simulink model "Test_CommSM"  (R2017b)
settings: Solver=VariableStepAuto  StartTime=0.0  StopTime=inf  RelTol=1e-3
model workspace (MAT data in the model file):
  AP = Simulink.Signal
  AP.DataType = 'double'
  AP.Dimensions = 1
  AP.DimensionsMode = 'auto'
  AP.Complexity = 'real'
  AP.SampleTime = -1
  AP.SamplingMode = 'auto'
  AP.InitialValue = '0'
  ZPT_1 = Simulink.Signal
  ZPT_1.DataType = 'double'
  ZPT_1.Dimensions = [1 3]
  ZPT_1.DimensionsMode = 'Fixed'
  ZPT_1.Complexity = 'real'
  ZPT_1.SampleTime = -1
  ZPT_1.SamplingMode = 'auto'
  ZPT_1.InitialValue = 'zeros(1,3)'
  ZZPT_1 = Simulink.Signal
  ZZPT_1.DataType = 'double'
  ZZPT_1.Dimensions = [3 4]
  ZZPT_1.DimensionsMode = 'Fixed'
  ZZPT_1.Complexity = 'real'
  ZZPT_1.SampleTime = -1
  ZZPT_1.SamplingMode = 'auto'
  ZZPT_1.InitialValue = 'zeros(3,4)'
settings Model: Creator=张紫薇  LastModifiedBy=张紫薇

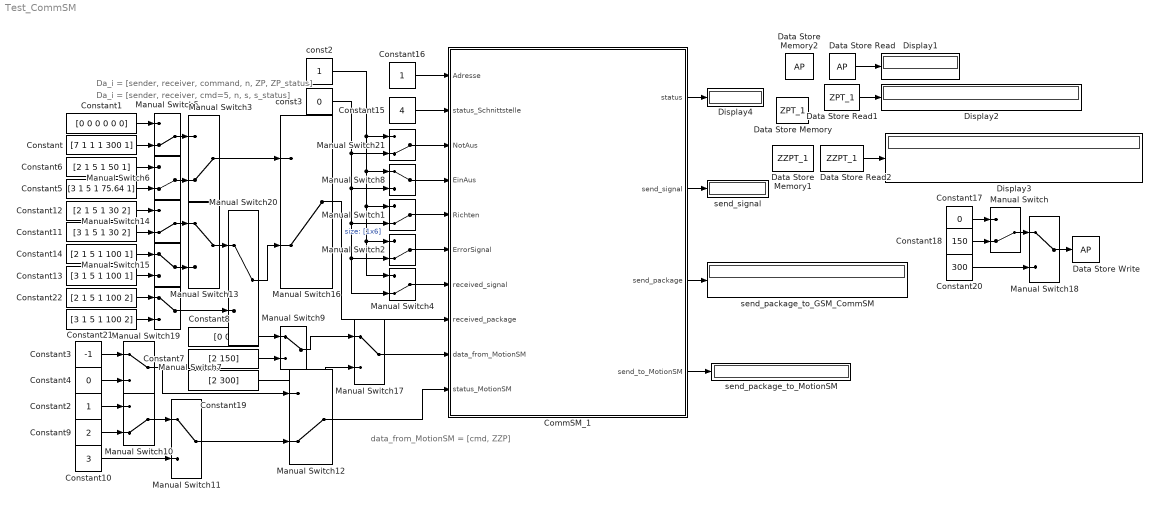
== system Test_CommSM ==
  note: data_from_MotionSM = [cmd, ZZP]
  note: Da_i = [sender, receiver, command, n, ZP, ZP_status]
  note: Da_i = [sender, receiver, cmd=5, n, s, s_status]
  CommSM_1 : Subsystem
  Constant : Constant  Value=[7 1 1 1 300 1]  OutDataTypeStr=double
  Constant1 : Constant  Value=[0 0 0 0 0 0]  OutDataTypeStr=double
  Constant10 : Constant  Value=3  OutDataTypeStr=double
  Constant11 : Constant  Value=[3 1 5 1 30 2]  OutDataTypeStr=double
  Constant12 : Constant  Value=[2 1 5 1 30 2]  OutDataTypeStr=double
  Constant13 : Constant  Value=[3 1 5 1 100 1]  OutDataTypeStr=double
  Constant14 : Constant  Value=[2 1 5 1 100 1]  OutDataTypeStr=double
  Constant15 : Constant  Value=4  OutDataTypeStr=double
  Constant16 : Constant
  Constant17 : Constant  Value=0  OutDataTypeStr=double
  Constant18 : Constant  Value=150  OutDataTypeStr=double
  Constant19 : Constant  Value=[2 300]  OutDataTypeStr=double
  Constant2 : Constant  OutDataTypeStr=double
  Constant20 : Constant  Value=300  OutDataTypeStr=double
  Constant21 : Constant  Value=[3 1 5 1 100 2]  OutDataTypeStr=double
  Constant22 : Constant  Value=[2 1 5 1 100 2]  OutDataTypeStr=double
  Constant3 : Constant  Value=-1  OutDataTypeStr=double
  Constant4 : Constant  Value=0  OutDataTypeStr=double
  Constant5 : Constant  Value=[3 1 5 1 75.64 1]  OutDataTypeStr=double
  Constant6 : Constant  Value=[2 1 5 1 50 1]  OutDataTypeStr=double
  Constant7 : Constant  Value=[2 150]  OutDataTypeStr=double
  Constant8 : Constant  Value=[0 0]  OutDataTypeStr=double
  Constant9 : Constant  Value=2  OutDataTypeStr=double
  Data Store Memory : DataStoreMemory  DataStoreName=ZPT_1  ReadBeforeWriteMsg=warning  WriteAfterWriteMsg=warning  WriteAfterReadMsg=warning  InitialValue=zeros(1,3)  ShowAdditionalParam=off  OutDataTypeStr=double  Dimensions=[1,3]
  Data Store Memory1 : DataStoreMemory  DataStoreName=ZZPT_1  ReadBeforeWriteMsg=warning  WriteAfterWriteMsg=warning  WriteAfterReadMsg=warning  InitialValue=zeros(3,4)  ShowAdditionalParam=off  OutDataTypeStr=double  Dimensions=[3,4]
  Data Store Memory2 : DataStoreMemory  DataStoreName=AP  ReadBeforeWriteMsg=warning  WriteAfterWriteMsg=warning  WriteAfterReadMsg=warning  ShowAdditionalParam=off  OutDataTypeStr=double  Dimensions=1
  Data Store Read : DataStoreRead  DataStoreName=AP
  Data Store Read1 : DataStoreRead  DataStoreName=ZPT_1
  Data Store Read2 : DataStoreRead  DataStoreName=ZZPT_1
  Data Store Write : DataStoreWrite  DataStoreName=AP
  Display{1..4} (4 alike) : Display
  Manual Switch{,1..6,10,12,14,16,21} (12 alike) : ManualSwitch  CurrentSetting=0
  Manual Switch{7..9,11,13,15,17..20} (10 alike) : ManualSwitch
  const2 : Constant  OutDataTypeStr=boolean
  const3 : Constant  Value=0  OutDataTypeStr=boolean
  send_package_to_GSM_CommSM : Display
  send_package_to_MotionSM : Display
  send_signal : Display
  wires:
  const2/1 -> Manual Switch4/1, Manual Switch2/1, Manual Switch1/1, Manual Switch8/1, Manual Switch21/1
  const3/1 -> Manual Switch21/2, Manual Switch4/2, Manual Switch2/2, Manual Switch1/2, Manual Switch8/2
  Manual Switch21/1 -> CommSM_1/3(NotAus)
  Manual Switch8/1 -> CommSM_1/4(EinAus)
  Manual Switch1/1 -> CommSM_1/5(Richten)
  Manual Switch2/1 -> CommSM_1/6(ErrorSignal)
  Manual Switch4/1 -> CommSM_1/7(received_signal)
  Manual Switch5/1 -> Manual Switch3/1
  Constant1/1 -> Manual Switch5/1
  Constant/1 -> Manual Switch5/2
  Constant6/1 -> Manual Switch6/1
  Constant5/1 -> Manual Switch6/2
  Manual Switch6/1 -> Manual Switch3/2
  Constant8/1 -> Manual Switch9/1
  Constant7/1 -> Manual Switch9/2
  Constant3/1 -> Manual Switch7/1
  Constant4/1 -> Manual Switch7/2
  Constant2/1 -> Manual Switch10/1
  Constant9/1 -> Manual Switch10/2
  Manual Switch10/1 -> Manual Switch11/1
  Constant10/1 -> Manual Switch11/2
  Manual Switch7/1 -> Manual Switch12/1
  Manual Switch11/1 -> Manual Switch12/2
  Manual Switch12/1 -> CommSM_1/10(status_MotionSM)
  Constant13/1 -> Manual Switch15/2
  Constant14/1 -> Manual Switch15/1
  Constant12/1 -> Manual Switch14/1
  Constant11/1 -> Manual Switch14/2
  Manual Switch14/1 -> Manual Switch13/1
  Manual Switch15/1 -> Manual Switch13/2
  Manual Switch3/1 -> Manual Switch16/1
  Manual Switch16/1 -> CommSM_1/8(received_package)  "size: [1x6]"
  CommSM_1/2(send_signal) -> send_signal/1
  CommSM_1/3(send_package) -> send_package_to_GSM_CommSM/1
  CommSM_1/4(send_to_MotionSM) -> send_package_to_MotionSM/1
  Constant15/1 -> CommSM_1/2(status_Schnittstelle)
  Constant16/1 -> CommSM_1/1(Adresse)
  CommSM_1/1(status) -> Display4/1
  Data Store Read2/1 -> Display3/1
  Data Store Read/1 -> Display1/1
  Data Store Read1/1 -> Display2/1
  Constant17/1 -> Manual Switch/1
  Constant18/1 -> Manual Switch/2
  Constant19/1 -> Manual Switch17/2
  Manual Switch9/1 -> Manual Switch17/1
  Manual Switch17/1 -> CommSM_1/9(data_from_MotionSM)
  Constant20/1 -> Manual Switch18/2
  Manual Switch/1 -> Manual Switch18/1
  Manual Switch18/1 -> Data Store Write/1
  Constant22/1 -> Manual Switch19/1
  Constant21/1 -> Manual Switch19/2
  Manual Switch19/1 -> Manual Switch20/2
  Manual Switch13/1 -> Manual Switch20/1
  Manual Switch20/1 -> Manual Switch16/2

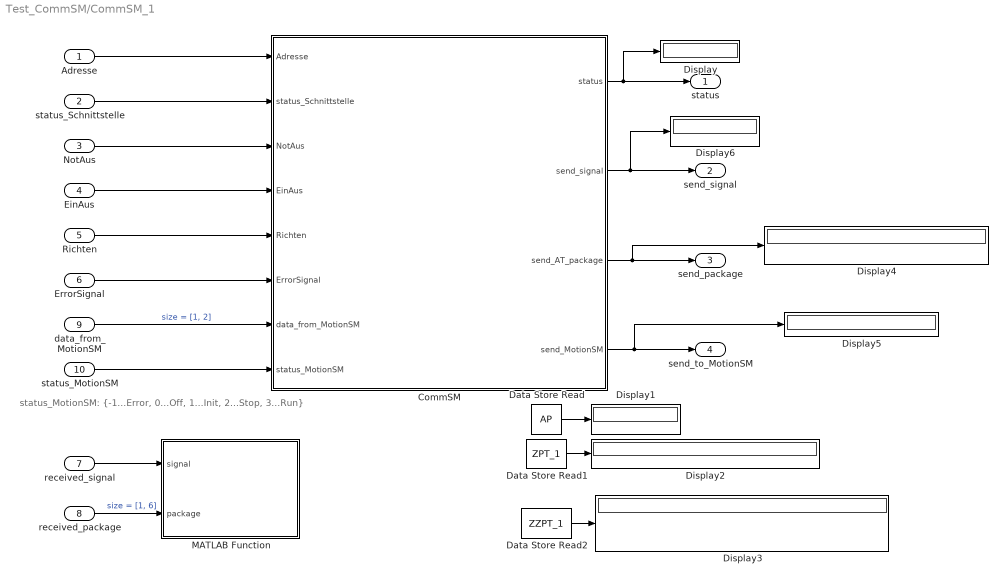
== system Test_CommSM/CommSM_1 ==
  note: status_MotionSM: {-1...Error, 0...Off, 1...Init, 2...Stop, 3...Run}
  Adresse : Inport  OutDataTypeStr=double  PortDimensions=1
  status_Schnittstelle : Inport  Port=2  OutDataTypeStr=double  PortDimensions=1
  NotAus : Inport  Port=3  OutDataTypeStr=boolean  PortDimensions=1
  EinAus : Inport  Port=4  OutDataTypeStr=boolean  PortDimensions=1
  Richten : Inport  Port=5  OutDataTypeStr=boolean  PortDimensions=1
  ErrorSignal : Inport  Port=6  OutDataTypeStr=boolean  PortDimensions=1
  received_signal : Inport  Port=7  OutDataTypeStr=boolean  PortDimensions=1
  received_package : Inport  Port=8  OutDataTypeStr=double  PortDimensions=6
  data_from_MotionSM : Inport  Port=9  OutDataTypeStr=double  PortDimensions=2
  status_MotionSM : Inport  Port=10  OutDataTypeStr=double  PortDimensions=1
  CommSM : Stateflow chart  TreatAsAtomicUnit=on
  Data Store Read : DataStoreRead  DataStoreName=AP
  Data Store Read1 : DataStoreRead  DataStoreName=ZPT_1
  Data Store Read2 : DataStoreRead  DataStoreName=ZZPT_1
  Display{,1..6} (7 alike) : Display
  MATLAB Function : MATLAB Function  TreatAsAtomicUnit=on
  status : Outport  OutDataTypeStr=double  PortDimensions=1
  send_signal : Outport  Port=2  OutDataTypeStr=boolean  PortDimensions=1
  send_package : Outport  Port=3  OutDataTypeStr=double  PortDimensions=6
  send_to_MotionSM : Outport  Port=4  OutDataTypeStr=double  PortDimensions=2
  wires:
  NotAus/1 -> CommSM/3(NotAus)
  EinAus/1 -> CommSM/4(EinAus)
  Richten/1 -> CommSM/5(Richten)
  ErrorSignal/1 -> CommSM/6(ErrorSignal)
  status_Schnittstelle/1 -> CommSM/2(status_Schnittstelle)
  received_signal/1 -> MATLAB Function/1(signal)
  received_package/1 -> MATLAB Function/2(package)  "size = [1, 6]"
  data_from_MotionSM/1 -> CommSM/7(data_from_MotionSM)  "size = [1, 2]"
  status_MotionSM/1 -> CommSM/8(status_MotionSM)
  Adresse/1 -> CommSM/1(Adresse)
  CommSM/1(status) -> Display/1, status/1
  CommSM/3(send_AT_package) -> Display4/1, send_package/1
  CommSM/4(send_MotionSM) -> Display5/1, send_to_MotionSM/1
  CommSM/2(send_signal) -> Display6/1, send_signal/1
  Data Store Read/1 -> Display1/1
  Data Store Read1/1 -> Display2/1
  Data Store Read2/1 -> Display3/1

== matlab function Test_CommSM/CommSM_1/MATLAB Function ==
  data: signal input boolean size=1; package input double size=[1,6]; ZPT_1 data_store_memory; ZZPT_1 data_store_memory
%Protokoll
%SummenTelegramm = [HDR, SDT, END]
	%HDR: header,	SDT: Summen-Daten-Telegramm,    END: Ender

%SDT = [SDT_7, SDT_1, SDT_2, SDT_3]
%SDT_i = [Da_i, De_i]
	%Da: Data, De: Delay
	%i...{1,2,3,7}	%7...GSM, 1-3...CommSM1-3

%Da_i = [sender, receiver, cmd, N, ZP, ZP_status]
	%sender,receiver...{1,2,3,7,255}	%255...Broadcast
	%cmd: 1...addP, 2...getP, 3...setS, 4...getS
	%ZP_status: 0...none, 1...wait, 2...active, 3...done, 4...error

%Da_i = [sender, receiver, cmd, N, s, s_status]
	%cmd: 5...negO
	%s_status: 0...none, 1...negotiation, 2...excute, 3...done

function receive_AT(signal, package)

global ZPT_1
global ZZPT_1

if signal
    switch package(1)  % from GSM
        case 7
            if (package(3) == 1)   % add Position
                if ZPT_1(1) == 0
                    ZPT_1 = package(4:6)';    %[n, ZP, status='wait']
                end
            end
            
        case {2,3}      % from CommSM_2 or CommSM_3
            if package(3) == 5      % negotiation
                switch package(6)
                    case 1      % nego
                        ZZPT_1(package(1),:) = [package(4), 0, package(5:6)];     % [n, ZP, s%, status='nego']
                    case 2      % excu
                        if ZZPT_1(package(1),4) == 1
                            ZZPT_1(package(1),4) = package(6);
                        end
                end
            end
    end
end

end

== stateflow chart Test_CommSM/CommSM_1/CommSM ==
  state Init
    entry: 	status=1;
    send_AT_package=[Adresse, zeros(1,5)];
    send_signal=false;
    send_MotionSM=[0,0];
  state Aus
    entry: status=0;
  state Ein
    note: % Protokoll
        | % SummenTelegramm = [HDR, SDT, END]
        | %HDR: header, SDT: Summen-Daten-Telegramm, END: Ender
        |
        | % SDT = [SDT_7, SDT_1, SDT_2, SDT_3]
        | % SDT_i = [Da_i, De_i]
        | %Da: Data, De: Delay
        | %i...{1,2,3,7} %7...GSM, 1-3...CommSM1-3
        |
        | % Da_i = [sender, receiver, cmd, N, ZP, ZP_status]
        | %sender,receiver...{1,2,3,7,255} %255...Broadcast
        | %cmd: 1...addP, 2...getP, 3...setS, 4...getS
        | %ZP_status: 0...none, 1...wait, 2...active, 3...done, 4...error
        |
        | % Da_i = [sender, receiver, cmd, N, s , s _status]
        | %cmd: 5 ...negO
        | % s _status: 0...none, 1...negotiation, 2...excute, 3...done
    state Free
      entry:	status=2;
      send_signal=false;
      send_AT_package=zeros(1,6);
    state SkillRequest
      entry:	status=3;
      send_AT_package=[Adresse, 7, 2, ZPT_1(1), ZPT_1(2), ZPT_1(3)];
      % AT=[CommSM, GSM, getP, n, ZP, wait];
      send_signal=true;
    state send_AT_2_GSM
      entry:	status=13;
      send_AT_package=[Adresse, 7, 3, ZPT_1(1), ZPT_1(2), ZPT_1(3)];
      %AT=[CommSM, GSM, setS, n, ZP, done];
      send_signal=true;
    state activ
      entry:	status=4;
      ZPT_1(3)=2;	% status='active'
      send_AT_package=[Adresse, 7, 3, ZPT_1(1), ZPT_1(2), ZPT_1(3)];
      % AT=[CommSM, GSM, setS, n, ZP, activ];
      send_signal=true;
    state Arrival
      entry:	status=12;
      ZPT_1(3)=3;
    state check_ZP
      entry: 	status=5;
      s=checkZP(ZZP_old, Adresse);
      % s-range: [0, 100], ZZP_old: ZZP for last Loop
      send_AT_package=[Adresse, 255, 5, ZPT_1(1), s, 1];
      % AT=[CommSM, Broadcast, negO, n, s, nego];
      send_signal=true;
    state MotionSM
      entry:	status=11;
      send_MotionSM=[3, ZZPT_1(Adresse,2)];	%excute ZZP
    state Nego_wait
      entry: 	status=6;
    state Wait_excution
      entry:	status=10;
      send_AT_package=[Adresse, 255, 5, ZPT_1(1), ZZPT_1(Adresse, 4), 2];
      %AT=[CommSM, Broadcast, negO, n, s, excu];
      send_signal=true;
      send_MotionSM=[1, ZZPT_1(Adresse,2)]; %set ZZP
    state status_excution
      entry: 	status=9;
      ZZPT_1(Adresse,4)=2; %excu
    state s_Compair
      entry: 	status=7; s_new=s_compair(Adresse);
    state ZZP_new
      entry:	status=8;
      ZZPT_1(Adresse,3)=s_new;
      ZZPT_1(Adresse,2)=AP+(ZPT_1(2)-AP)*(s_new/100);
    (default) -> Free
    (junction 230) -> Free
    send_AT_2_GSM -> (junction 230) : {send_signal=false; ZPT_1=zeros(1,3)';}
    Free -> SkillRequest : %Datei von GSM empfangen
        | [ZPT_1(1)~=0]
    SkillRequest -> activ : %status="wait" && MotionSM kein Fehler
        | [ZPT_1(3)==1 && status_MotionSM>=1]{send_signal=false;}
    (junction 231) -> send_AT_2_GSM
    Arrival -> (junction 231)
    (junction 228) -> (junction 231)
    MotionSM -> Arrival [order 1] : % ZP == ZZP -> wait until ZP == AP
        | [ZPT_1(2)==AP && ZZPT_1(Adresse,2)==AP && status_MotionSM ==2]
        | {ZZPT_1=zeros(3,4); send_MotionSM=zeros(1,2)}
    activ -> (junction 232) : [ZPT_1(3)==2]{send_signal=false;}
    (junction 233) -> (junction 232)
    (junction 232) -> check_ZP
    MotionSM -> (junction 233) [order 2] : % ZP~=ZZP = ZZP = ZZP -> cycle
        | [ZPT_1(2)~=ZZPT_1(Adresse,2)]
        | {ZZP_old=ZZPT_1(Adresse,2); ZZPT_1=zeros(3,4);}
    (junction 254) -> MotionSM : [status_MotionSM==2] % Motor stoped
    check_ZP -> Nego_wait : {s=0; send_signal=false;}
    (junction 229) -> (junction 254) : % ZZP received from MotionSM
        | [data_from_MotionSM(1)==2 && data_from_MotionSM(2)==ZZPT_1(Adresse,2)]{ZZP_old=0;}
    Wait_excution -> (junction 229) : [ZZPT_1(1,4)==2 && ZZPT_1(2,4)==2 && ZZPT_1(3,4)==2]{send_signal=false;}
    Nego_wait -> (junction 228) [order 1] : [ZPT_1(3)==3] % ZP = AP
    Nego_wait -> (junction 227) [order 2] : [ZPT_1(3)==2] % ZP "activ"
    status_excution -> Wait_excution : [status_MotionSM>=2]  % 2 or 3
    (junction 227) -> s_Compair : %ZZPT erfüllt
        | [ZZPT_1(1,1)==1 && ZZPT_1(2,1)==1 && ZZPT_1(3,1)==1 && ZZPT_1(1,1)~=0]
    s_Compair -> (junction 205)
    (junction 200) -> status_excution : {s_new=0;}
    (junction 205) -> (junction 200) [order 2] : [s_new>=ZZPT_1(Adresse,3)]
    (junction 205) -> ZZP_new [order 1] : [s_new<ZZPT_1(Adresse,3)]
    ZZP_new -> (junction 200)
  state Error
    entry: status=-1;
  (default) -> Aus
  Aus -> Init : [EinAus && ~NotAus && ~ErrorSignal]
  Init -> Aus [order 1] : [~EinAus]
  Init -> Error [order 2] : [NotAus]
  Error -> Aus [order 1] : [~EinAus]
  Ein -> Aus [order 1] : [~EinAus]
  Error -> Init [order 2] : [Richten && ~NotAus && ~ErrorSignal]
  Init -> Ein [order 3] : [status_Schnittstelle==4]{send_signal=false;}
  Ein -> Error [order 2] : [NotAus]
  data: zzp_old function_input double size=1; S function_output; adress function_input double size=1; S_new function_output double size=1; nr function_input double size=1; Adresse input double size=1; status_Schnittstelle input double size=1; NotAus input boolean size=1; EinAus input boolean size=1; Richten input boolean size=1; ErrorSignal input boolean size=1; status output double size=1; send_signal output boolean size=1 =false; send_AT_package output double size=[1,6] =zeros(1,6); data_from_MotionSM input double size=[1,2]; status_MotionSM input double size=1; ZPT_1 data_store_memory; ZZPT_1 data_store_memory; AP data_store_memory; s local double size=1 =0; s_new local double size=1 =0; send_MotionSM output double size=[1,2] =zeros(1,2); ZZP_old local double size=1 =0
  function S = checkZP(zzp_old, adress):
    | %ZPT_1 = [ZP_Nr., ZP, status]
    | %status: {0...none, 1...wait, 2...active, 3...done, 4...error}
    | 
    | %ZZPT_1(CommSM_i,:) = [ZP-Nr., ZZP, s%, status]
    | %status: {0...none, 1...negotiation, 2...excution, 3...done}
    | 
    | function S = checkZP(zzp_old, adress)
    | %1. prüfen, ob ZP unter begrenzte Bedienung erreichbar ist
    |         %Ja     --> ZZP = ZP
    |         %Nein   --> neuen ZZP erzeugen
    | %2. neu ausgerechnete ZZP in der ZZP Tabelle einschreiben
    |  
    | global AP
    | global ZPT_1
    | global ZZPT_1
    | 
    | a_max = 1000;   % mm/s^2
    | v_max = 1000;   % mm/s
    | d_T = 10;    % s
    | 
    | s_max = a_max*d_T*d_T/4;
    | if zzp_old <= 0             %last ZZP to arrive. After the Motor is started, ZZP_old = ZZP, ZZPT = zeros(3,4);
    |     s0 = ZPT_1(2) - AP;     %ZP - AP
    | else
    |     s0 = ZPT_1(2) - zzp_old;    %excist last ZZP
    | end
    | 
    | if abs(s0) <= s_max
    |     S = 100;                    % 100% erreichbar
    | elseif abs(s0) > 0 && abs(s0) < 100
    |     S = abs(100*s_max/s0);      % s% s: [0, 100]
    |     S = fix(1000*S)/1000;       % Genauigkeit = 10000*0.001%=0.1 mm
    | else
    |     S = 0;                      % ZP = AP, Achse keine Bewegung
    | end
    | 
    | %ZZP-Tabelle erfüllen
    | if zzp_old <= 0
    |     ZZP_new = AP + s0*S/100;        %neue ZZP in der ZZP-Tabelle einschreiben
    | else
    |     ZZP_new = zzp_old+s0*S/100;
    | end
    | 
    | if S == 0
    |     %ZZPT_1(nr,:) = [ZPT_1(1), ZZP_new, s, 3];
    |     ZPT_1(3) = 3;
    | else
    |     ZZPT_1(adress,:) = [ZPT_1(1), ZZP_new, S, 1];
    | end
    | 
    | end
  function S_new = s_compair(nr):
    | function S_new = s_compair(nr)
    | 
    | global ZZPT_1
    | 
    | s_ = ZZPT_1(:,3);
    | 
    | S_new = s_(nr);          % CommSM_me
    | 
    | for i = 1:3                         % s==0 --> s=100
    |     if i ~= nr && s_(i)== 0
    |         s_(i) = 100;
    |     end
    | end
    | 
    | s_min = min(s_);
    | if S_new > s_min
    |     S_new = s_min;
    | end
    | 
    | end
